simulink model "test_duc"  (R2015a)
settings: Solver=ode45  StartTime=0.0  StopTime=16*4100  RelTol=1e-3
libraries: xbsIndex_r4 x14, simulink x2
settings Model: CovSFcnEnable=off  Creator=alexp  LastModifiedBy=alexp
settings DebuggingCC: SolverPrmCheckMsg=warning

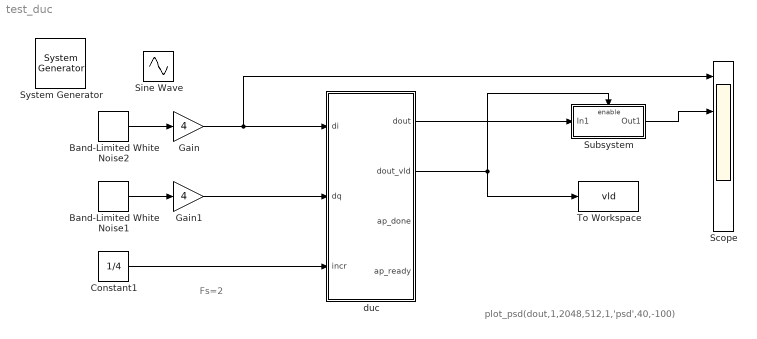
== system test_duc ==
  note: Fs=2
  note: plot_psd(dout,1,2048,512,1,'psd',40,-100)
  " System Generator" : xbsIndex_r4/ System Generator  Tag=genX  xilinxfamily=zynq  part=xc7z020  speed=-1  package=clg484  synthesis_tool=Vivado  clock_wrapper=Clock Enables  directory=./netlist  proj_type=Vivado  Synth_file=Vivado Synthesis Defaults  Impl_file=Vivado Implementation Defaults  testbench=off  simulink_period=1  sysclk_period=5  dcm_input_clock_period=10  incr_netlist=off  trim_vbits=Everywhere in SubSystem  dbl_ovrd=According to Block Masks  core_generation=According to Block Masks  run_coregen=off  deprecated_control=off  eval_field=0  block_type=sysgen
  Band-Limited White Noise1 : simulink/Sources/Band-Limited White Noise  Cov=[0.1]  Ts=16  seed=[1]
  Band-Limited White Noise2 : simulink/Sources/Band-Limited White Noise  Cov=[0.1]  Ts=16  seed=[2]
  Constant1 : Constant  Value=1/4  SampleTime=16
  Gain : Gain  Gain=4
  Gain1 : Gain  Gain=4
  Scope : Scope  NumInputPorts=5
      settings: YMin=-5~-5~-5~-5~-5  YMax=5~5~5~5~5
  Sine Wave : Sin  SineType=Sample based  Amplitude=1.99  Samples=32  SampleTime=16
  Subsystem : Subsystem
  To Workspace : ToWorkspace  VariableName=vld  SaveFormat=Structure  SampleTime=1
  duc : Subsystem
  wires:
  Band-Limited White Noise2/1 -> Gain/1
  Band-Limited White Noise1/1 -> Gain1/1
  duc/1(dout) -> Subsystem/1(In1)
  duc/2("dout_vld ") -> To Workspace/1, Subsystem/Enable
  Subsystem/1(Out1) -> Scope/2
  Constant1/1 -> duc/3(incr)
  Gain/1 -> duc/1(di), Scope/1
  Gain1/1 -> duc/2(dq)

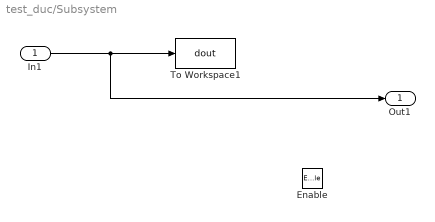
== system test_duc/Subsystem ==
  In1 : Inport
  Enable : EnablePort
  To Workspace1 : ToWorkspace  VariableName=dout  SampleTime=1
  Out1 : Outport
  wires:
  In1/1 -> Out1/1, To Workspace1/1

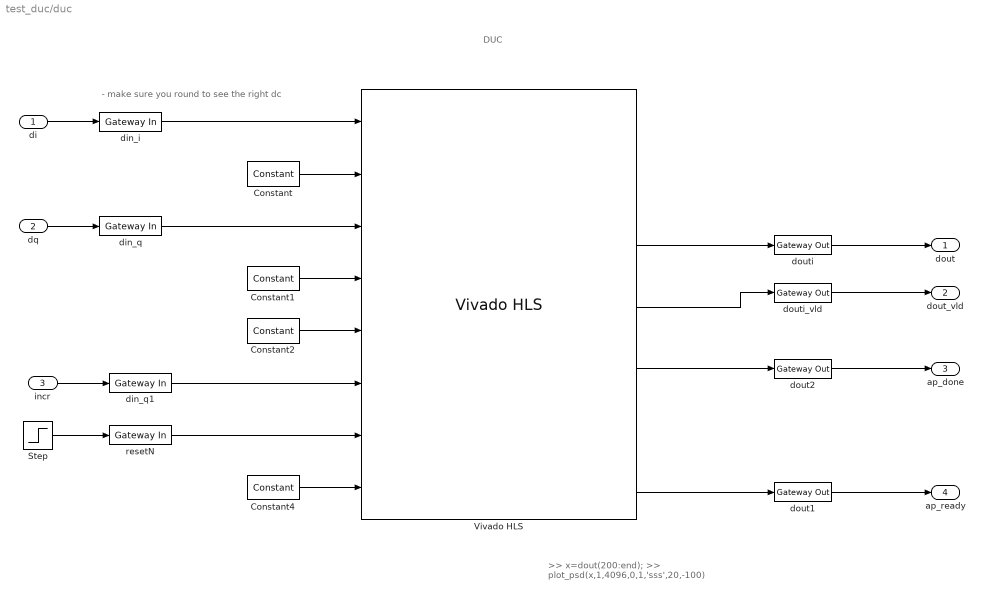
== system test_duc/duc ==
  note: DUC
  note: >> x=dout(200:end);
      | >> plot_psd(x,1,4096,0,1,'sss',20,-100)
  note: - make sure you round to see the right dc
  di : Inport
  dq : Inport  Port=2
  incr : Inport  Port=3
  Constant{,1..2,4} (4 alike) : xbsIndex_r4/Constant  const=1  gui_display_data_type=Boolean  arith_type=Boolean  n_bits=16  bin_pt=14  preci_type=Single  exp_width=8  frac_width=24  explicit_period=on  period=1  equ=P=C  opselect=C  inp2=PCIN>>17  opr=+  inp1=P  carry=CIN  dbl_ovrd=off  block_type=constant
  Step : Step  Time=10  SampleTime=1
  Vivado HLS : xbsIndex_r4/Vivado HLS  anytable='D:/design_QAM/duc_with_DDS/proj/sol2_b'  fast_sim=on  display_datatype=on  rate_propagation_method=Simulink system period  model_file_path=''  latency=1  block_type=hls
      settings: infoedit=This block allows including C,C++ and SystemC source files in System Generator for DSP designs.
  din_i : xbsIndex_r4/Gateway In  gui_display_data_type=Fixed-point  arith_type="Signed  (2's comp)"  n_bits=24  bin_pt=14  preci_type=Single  exp_width=8  frac_width=24  rows=1  columns=1  quantization="Round  (unbiased: +/- Inf)"  overflow=Wrap  period=1  UseAsADC=off  ADCChannel='1'  interface=None  automatic_assignment=on  address_offset=hex2dec('00')  intf_name=''  intf_description=''  timing_constraint=None  locs_specified=off  LOCs={}  io_standard={}  inherit_from_input=off  hdl_port=on  dbl_ovrd=off  block_type=gatewayin
  din_q : xbsIndex_r4/Gateway In  gui_display_data_type=Fixed-point  arith_type="Signed  (2's comp)"  n_bits=24  bin_pt=14  preci_type=Single  exp_width=8  frac_width=24  rows=1  columns=1  quantization="Round  (unbiased: +/- Inf)"  overflow=Wrap  period=1  UseAsADC=off  ADCChannel='1'  interface=None  automatic_assignment=on  address_offset=hex2dec('00')  intf_name=''  intf_description=''  timing_constraint=None  locs_specified=off  LOCs={}  io_standard={}  inherit_from_input=off  hdl_port=on  dbl_ovrd=off  block_type=gatewayin
  din_q1 : xbsIndex_r4/Gateway In  gui_display_data_type=Fixed-point  arith_type="Signed  (2's comp)"  n_bits=32  bin_pt=31  preci_type=Single  exp_width=8  frac_width=24  rows=1  columns=1  quantization="Round  (unbiased: +/- Inf)"  overflow=Wrap  period=1  UseAsADC=off  ADCChannel='1'  interface=None  automatic_assignment=on  address_offset=hex2dec('00')  intf_name=''  intf_description=''  timing_constraint=None  locs_specified=off  LOCs={}  io_standard={}  inherit_from_input=off  hdl_port=on  dbl_ovrd=off  block_type=gatewayin
  dout1 : xbsIndex_r4/Gateway Out  inherit_from_input=off  hdl_port=on  rows=1  columns=1  UseAsDAC=off  DACChannel='1'  interface=None  automatic_assignment=on  address_offset=hex2dec('00')  intf_name=''  intf_description=''  timing_constraint=None  locs_specified=off  LOCs={}  io_standard={}  block_type=gatewayout
  dout2 : xbsIndex_r4/Gateway Out  inherit_from_input=off  hdl_port=on  rows=1  columns=1  UseAsDAC=off  DACChannel='1'  interface=None  automatic_assignment=on  address_offset=hex2dec('00')  intf_name=''  intf_description=''  timing_constraint=None  locs_specified=off  LOCs={}  io_standard={}  block_type=gatewayout
  douti : xbsIndex_r4/Gateway Out  inherit_from_input=off  hdl_port=on  rows=1  columns=1  UseAsDAC=off  DACChannel='1'  interface=None  automatic_assignment=on  address_offset=hex2dec('00')  intf_name=''  intf_description=''  timing_constraint=None  locs_specified=off  LOCs={}  io_standard={}  block_type=gatewayout
  douti_vld : xbsIndex_r4/Gateway Out  inherit_from_input=off  hdl_port=on  rows=1  columns=1  UseAsDAC=off  DACChannel='1'  interface=None  automatic_assignment=on  address_offset=hex2dec('00')  intf_name=''  intf_description=''  timing_constraint=None  locs_specified=off  LOCs={}  io_standard={}  block_type=gatewayout
  resetN : xbsIndex_r4/Gateway In  gui_display_data_type=Boolean  arith_type=Boolean  n_bits=16  bin_pt=0  preci_type=Single  exp_width=8  frac_width=24  rows=1  columns=1  quantization=Truncate  overflow=Wrap  period=1  UseAsADC=off  ADCChannel='1'  interface=None  automatic_assignment=on  address_offset=hex2dec('00')  intf_name=''  intf_description=''  timing_constraint=None  locs_specified=off  LOCs={}  io_standard={}  inherit_from_input=off  hdl_port=on  dbl_ovrd=off  block_type=gatewayin
  dout : Outport
  "dout_vld " : Outport  Port=2
  ap_done : Outport  Port=3
  ap_ready : Outport  Port=4
  wires:
  Step/1 -> resetN/1
  din_i/1 -> Vivado HLS/1
  di/1 -> din_i/1
  Constant2/1 -> Vivado HLS/5
  Constant/1 -> Vivado HLS/2
  douti/1 -> dout/1
  dout2/1 -> ap_done/1
  dq/1 -> din_q/1
  resetN/1 -> Vivado HLS/7
  din_q1/1 -> Vivado HLS/6
  Constant4/1 -> Vivado HLS/8
  douti_vld/1 -> "dout_vld "/1
  dout1/1 -> ap_ready/1
  Vivado HLS/3 -> douti/1
  Vivado HLS/4 -> douti_vld/1
  Vivado HLS/5 -> dout2/1
  Vivado HLS/7 -> dout1/1
  incr/1 -> din_q1/1
  Constant1/1 -> Vivado HLS/4
  din_q/1 -> Vivado HLS/3
